simulink model "LDFIsys"  (R2023a)
settings: Solver=FixedStepDiscrete  StartTime=0.0  StopTime=cin.TimeInfo.End  RelTol=1e-3
values from neighbouring files (symbols this model uses):
  cmax = rows*cols    [LDFItest.m]    (also in LDXItest.m; LXFItest.m; LXFXtest.m; LXXItest.m)
  hmax = ceil((rows*cols/sqrt(12))/pow2(logDPS.stde,8-sbin))    [LDFItest.m]    (also in LDXItest.m; LXFItest.m; LXFXtest.m; LXXItest.m)
  sbin = 4    [LDFItest.m]    (also in LDXItest.m; LXFItest.m; LXFXtest.m; LXXItest.m)
  Ts = 1/(30*rows*cols)    [LDFItest.m]    (also in LDXItest.m; LXFItest.m; LXFXtest.m; LXXItest.m)
libraries: simulink x20, hdlsllib x5
settings Model: Creator=dileepan  LastModifiedBy=dileepan
settings DataIOCC: SaveOutput=off  SignalLogging=off  DSMLogging=off  SaveTime=off  ReturnWorkspaceOutputs=off

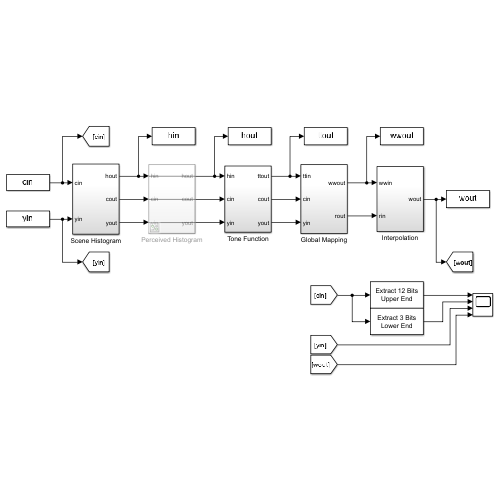
[thumbnail: Simulink's stored preview of the top-level diagram]
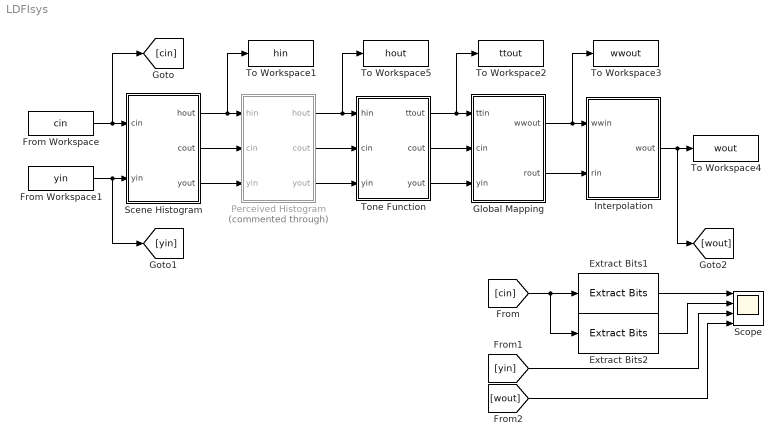
== system LDFIsys ==
  Extract Bits1 : simulink/Logic and Bit Operations/Extract Bits  bitsToExtract=Range starting with most significant bit  numBits=16-sbin  bitIdxRange=2+[0 15-sbin]  outScalingMode=Treat bit field as an integer
  Extract Bits2 : simulink/Logic and Bit Operations/Extract Bits  bitsToExtract=Range ending with least significant bit  numBits=3  bitIdxRange=[0 1]  outScalingMode=Treat bit field as an integer
  From Workspace : FromWorkspace  VariableName=cin  SampleTime=Ts  Interpolate=off  OutputAfterFinalValue=Setting to zero
  From Workspace1 : FromWorkspace  VariableName=yin  SampleTime=Ts  Interpolate=off  OutputAfterFinalValue=Setting to zero
  Global Mapping : Subsystem
  Interpolation : Subsystem
  Perceived Histogram : Subsystem  Commented=through
  Scene Histogram : Subsystem
  Scope : Scope  NumInputPorts=4
  To Workspace1 : ToWorkspace  VariableName=hin  SaveFormat=Timeseries  SampleTime=-1
      settings: Save2DSignal=2-D array (concatenate along first dimension)
  To Workspace2 : ToWorkspace  VariableName=ttout  SaveFormat=Timeseries  SampleTime=-1
      settings: Save2DSignal=2-D array (concatenate along first dimension)
  To Workspace3 : ToWorkspace  VariableName=wwout  SaveFormat=Timeseries  SampleTime=-1
      settings: Save2DSignal=2-D array (concatenate along first dimension)
  To Workspace4 : ToWorkspace  VariableName=wout  SaveFormat=Timeseries  SampleTime=-1
      settings: Save2DSignal=2-D array (concatenate along first dimension)
  To Workspace5 : ToWorkspace  VariableName=hout  SaveFormat=Timeseries  SampleTime=-1
      settings: Save2DSignal=2-D array (concatenate along first dimension)
  Tone Function : Subsystem
  wires:
  [cin] -> Extract Bits2/1, Extract Bits1/1
  Extract Bits1/1 -> Scope/1
  Extract Bits2/1 -> Scope/2
  [yin] -> Scope/3
  [wout] -> Scope/4
  Scene Histogram/3(yout) -> Perceived Histogram/3(yin)
  Scene Histogram/2(cout) -> Perceived Histogram/2(cin)
  Scene Histogram/1(hout) -> To Workspace1/1, Perceived Histogram/1(hin)
  Perceived Histogram/1(hout) -> To Workspace5/1, Tone Function/1(hin)
  Perceived Histogram/2(cout) -> Tone Function/2(cin)
  Perceived Histogram/3(yout) -> Tone Function/3(yin)
  Tone Function/1(ttout) -> To Workspace2/1, Global Mapping/1(ttin)
  Tone Function/2(cout) -> Global Mapping/2(cin)
  Tone Function/3(yout) -> Global Mapping/3(yin)
  Global Mapping/2(rout) -> Interpolation/2(rin)
  Global Mapping/1(wwout) -> To Workspace3/1, Interpolation/1(wwin)
  From Workspace/1 -> [cin], Scene Histogram/1(cin)
  Interpolation/1(wout) -> [wout], To Workspace4/1
  From Workspace1/1 -> [yin], Scene Histogram/2(yin)

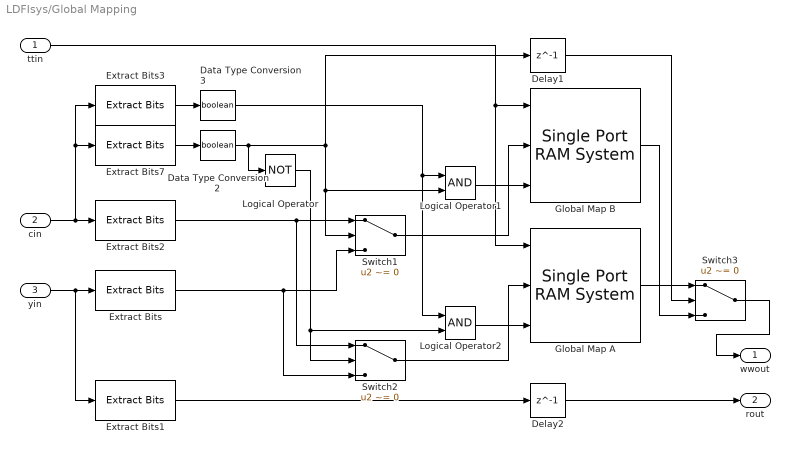
== system LDFIsys/Global Mapping ==
  ttin : Inport
  cin : Inport  Port=2
  yin : Inport  Port=3
  Data Type Conversion2 : DataTypeConversion  OutDataTypeStr=boolean  ConvertRealWorld=Stored Integer (SI)  SaturateOnIntegerOverflow=off  RndMeth=Floor
  Data Type Conversion3 : DataTypeConversion  OutDataTypeStr=boolean  ConvertRealWorld=Stored Integer (SI)  SaturateOnIntegerOverflow=off  RndMeth=Floor
  Delay1 : Delay  DelayLength=1
  Delay2 : Delay  DelayLength=1
  Extract Bits : simulink/Logic and Bit Operations/Extract Bits  bitsToExtract=Range starting with most significant bit  numBits=16-sbin  bitIdxRange=[0 7]  outScalingMode=Treat bit field as an integer
  Extract Bits1 : simulink/Logic and Bit Operations/Extract Bits  bitsToExtract=Range ending with least significant bit  numBits=sbin  bitIdxRange=0  outScalingMode=Treat bit field as an integer
  Extract Bits2 : simulink/Logic and Bit Operations/Extract Bits  bitsToExtract=Range starting with most significant bit  numBits=16-sbin  bitIdxRange=[2 17-sbin]  outScalingMode=Treat bit field as an integer
  Extract Bits3 : simulink/Logic and Bit Operations/Extract Bits  bitsToExtract=Range of bits  numBits=2  bitIdxRange=1  outScalingMode=Treat bit field as an integer
  Extract Bits7 : simulink/Logic and Bit Operations/Extract Bits  bitsToExtract=Range of bits  numBits=1  bitIdxRange=0  outScalingMode=Treat bit field as an integer
  Global Map A : hdlsllib/HDL RAMs/Single Port RAM System  RAMType=Single port  WriteOutputValue=New data  RAMInitialValue=0  SimulateUsing=Code generation
  Global Map B : hdlsllib/HDL RAMs/Single Port RAM System  RAMType=Single port  WriteOutputValue=New data  RAMInitialValue=0  SimulateUsing=Code generation
  Logical Operator : Logic  Operator=NOT  IconShape=distinctive  AllPortsSameDT=off  OutDataTypeStr=boolean
  Logical Operator1 : Logic  AllPortsSameDT=off  OutDataTypeStr=boolean
  Logical Operator2 : Logic  AllPortsSameDT=off  OutDataTypeStr=boolean
  Switch1 : Switch  Criteria=u2 ~= 0  SaturateOnIntegerOverflow=off  InputSameDT=off
  Switch2 : Switch  Criteria=u2 ~= 0  SaturateOnIntegerOverflow=off  InputSameDT=off
  Switch3 : Switch  Criteria=u2 ~= 0  SaturateOnIntegerOverflow=off  InputSameDT=off
  wwout : Outport
  rout : Outport  Port=2
  wires:
  yin/1 -> Extract Bits1/1, Extract Bits/1
  Extract Bits7/1 -> Data Type Conversion2/1
  Extract Bits/1 -> Switch2/3, Switch1/3
  Data Type Conversion3/1 -> Logical Operator1/1, Logical Operator2/1
  Switch1/1 -> Global Map B/2
  cin/1 -> Extract Bits2/1, Extract Bits3/1, Extract Bits7/1
  Extract Bits3/1 -> Data Type Conversion3/1
  Switch2/1 -> Global Map A/2
  Logical Operator/1 -> Logical Operator2/2, Switch2/2
  Extract Bits2/1 -> Switch2/1, Switch1/1
  Data Type Conversion2/1 -> Logical Operator/1, Delay1/1, Switch1/2, Logical Operator1/2
  Logical Operator1/1 -> Global Map B/3
  Logical Operator2/1 -> Global Map A/3
  Global Map A/1 -> Switch3/1
  Global Map B/1 -> Switch3/3
  ttin/1 -> Global Map B/1, Global Map A/1
  Extract Bits1/1 -> Delay2/1
  Delay2/1 -> rout/1
  Switch3/1 -> wwout/1
  Delay1/1 -> Switch3/2

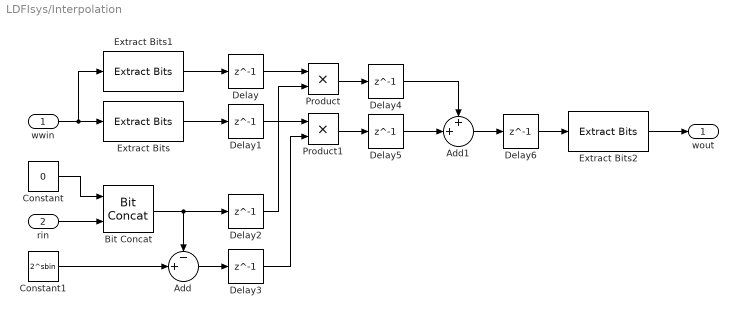
== system LDFIsys/Interpolation ==
  wwin : Inport
  rin : Inport  Port=2
  Add : Sum  Inputs=-+|  OutDataTypeStr=Inherit: Same as accumulator
  Add1 : Sum  Inputs=++|  OutDataTypeStr=Inherit: Same as accumulator
  Bit Concat : hdlsllib/Logic and Bit Operations/Bit Concat  numInputs=2
  Constant : Constant  Value=0  OutDataTypeStr=fixdt(0,1,0)  SampleTime=Ts
  Constant1 : Constant  Value=2^sbin  OutDataTypeStr=fixdt(0,sbin+1,0)  SampleTime=Ts
  Delay{,1..6} (7 alike) : Delay  DelayLength=1
  Extract Bits : simulink/Logic and Bit Operations/Extract Bits  bitsToExtract=Lower half  numBits=8  bitIdxRange=[0 7]  outScalingMode=Treat bit field as an integer
  Extract Bits1 : simulink/Logic and Bit Operations/Extract Bits  bitsToExtract=Upper half  numBits=8  bitIdxRange=[0 7]  outScalingMode=Treat bit field as an integer
  Extract Bits2 : simulink/Logic and Bit Operations/Extract Bits  bitsToExtract=Range of bits  numBits=8  bitIdxRange=[0 7]+sbin  outScalingMode=Treat bit field as an integer
  Product : Product  OutDataTypeStr=fixdt(0,8+sbin+1,0)
  Product1 : Product  OutDataTypeStr=fixdt(0,8+sbin+1,0)
  wout : Outport
  wires:
  wwin/1 -> Extract Bits1/1, Extract Bits/1
  rin/1 -> Bit Concat/2
  Constant/1 -> Bit Concat/1
  Extract Bits1/1 -> Delay/1
  Extract Bits/1 -> Delay1/1
  Bit Concat/1 -> Delay2/1, Add/1
  Delay2/1 -> Product/2
  Add/1 -> Delay3/1
  Delay3/1 -> Product1/2
  Delay/1 -> Product/1
  Delay1/1 -> Product1/1
  Product/1 -> Delay4/1
  Product1/1 -> Delay5/1
  Delay5/1 -> Add1/2
  Delay4/1 -> Add1/1
  Add1/1 -> Delay6/1
  Delay6/1 -> Extract Bits2/1
  Extract Bits2/1 -> wout/1
  Constant1/1 -> Add/2

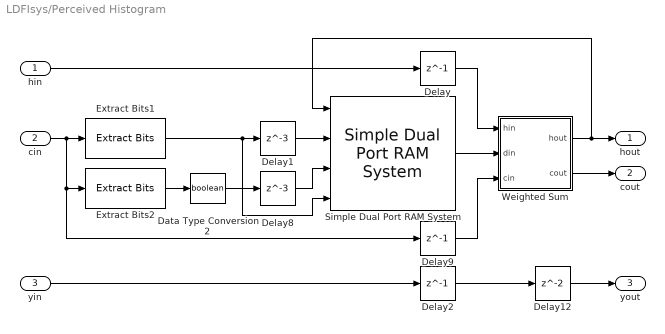
== system LDFIsys/Perceived Histogram ==
  hin : Inport
  cin : Inport  Port=2
  yin : Inport  Port=3
  Data Type Conversion2 : DataTypeConversion  OutDataTypeStr=boolean  ConvertRealWorld=Stored Integer (SI)  SaturateOnIntegerOverflow=off  RndMeth=Floor
  Delay : Delay  DelayLength=1
  Delay1 : Delay  DelayLength=3
  Delay12 : Delay
  Delay2 : Delay  DelayLength=1
  Delay8 : Delay  DelayLength=3
  Delay9 : Delay  DelayLength=1
  Extract Bits1 : simulink/Logic and Bit Operations/Extract Bits  bitsToExtract=Range starting with most significant bit  numBits=16-sbin  bitIdxRange=[3 18-sbin]  outScalingMode=Treat bit field as an integer
  Extract Bits2 : simulink/Logic and Bit Operations/Extract Bits  bitsToExtract=Range of bits  numBits=bitc  bitIdxRange=1  outScalingMode=Treat bit field as an integer
  Simple Dual Port RAM System : hdlsllib/HDL RAMs/Simple Dual Port RAM System  RAMType=Simple dual port  WriteOutputValue=New data  RAMInitialValue=0  SimulateUsing=Code generation
  Weighted Sum : Subsystem
  hout : Outport
  cout : Outport  Port=2
  yout : Outport  Port=3
  wires:
  hin/1 -> Delay/1
  Delay1/1 -> Simple Dual Port RAM System/2
  Extract Bits1/1 -> Simple Dual Port RAM System/4, Delay1/1
  cin/1 -> Delay9/1, Extract Bits2/1, Extract Bits1/1
  Delay8/1 -> Simple Dual Port RAM System/3
  yin/1 -> Delay2/1
  Delay12/1 -> yout/1
  Data Type Conversion2/1 -> Delay8/1
  Extract Bits2/1 -> Data Type Conversion2/1
  Simple Dual Port RAM System/1 -> Weighted Sum/2(din)
  Delay/1 -> Weighted Sum/1(hin)
  Delay9/1 -> Weighted Sum/3(cin)
  Delay2/1 -> Delay12/1
  Weighted Sum/1(hout) -> Simple Dual Port RAM System/1, hout/1
  Weighted Sum/2(cout) -> cout/1

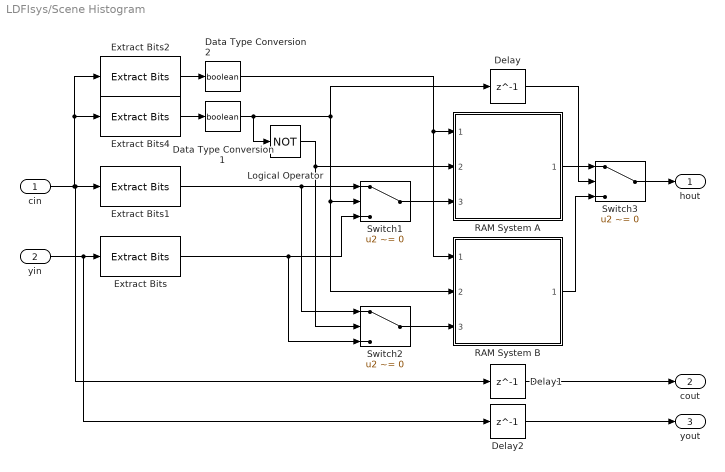
== system LDFIsys/Scene Histogram ==
  cin : Inport
  yin : Inport  Port=2
  Data Type Conversion1 : DataTypeConversion  OutDataTypeStr=boolean  ConvertRealWorld=Stored Integer (SI)  SaturateOnIntegerOverflow=off  RndMeth=Floor
  Data Type Conversion2 : DataTypeConversion  OutDataTypeStr=boolean  ConvertRealWorld=Stored Integer (SI)  SaturateOnIntegerOverflow=off  RndMeth=Floor
  Delay : Delay  DelayLength=1
  Delay1 : Delay  DelayLength=1
  Delay2 : Delay  DelayLength=1
  Extract Bits : simulink/Logic and Bit Operations/Extract Bits  bitsToExtract=Range starting with most significant bit  numBits=16-sbin  bitIdxRange=[0 7]  outScalingMode=Treat bit field as an integer
  Extract Bits1 : simulink/Logic and Bit Operations/Extract Bits  bitsToExtract=Range starting with most significant bit  numBits=16-sbin  bitIdxRange=[2 17-sbin]  outScalingMode=Treat bit field as an integer
  Extract Bits2 : simulink/Logic and Bit Operations/Extract Bits  bitsToExtract=Range of bits  numBits=2  bitIdxRange=1  outScalingMode=Treat bit field as an integer
  Extract Bits4 : simulink/Logic and Bit Operations/Extract Bits  bitsToExtract=Range of bits  numBits=1  bitIdxRange=0  outScalingMode=Treat bit field as an integer
  Logical Operator : Logic  Operator=NOT  IconShape=distinctive  AllPortsSameDT=off  OutDataTypeStr=boolean
  RAM System A : Subsystem  ReferencedSubsystem=RAMsys
  RAM System B : Subsystem  ReferencedSubsystem=RAMsys
  Switch1 : Switch  Criteria=u2 ~= 0  SaturateOnIntegerOverflow=off  InputSameDT=off
  Switch2 : Switch  Criteria=u2 ~= 0  SaturateOnIntegerOverflow=off  InputSameDT=off
  Switch3 : Switch  Criteria=u2 ~= 0  SaturateOnIntegerOverflow=off  InputSameDT=off
  hout : Outport
  cout : Outport  Port=2
  yout : Outport  Port=3
  wires:
  Extract Bits2/1 -> Data Type Conversion2/1
  Extract Bits/1 -> Switch2/3, Switch1/3
  yin/1 -> Delay2/1, Extract Bits/1
  Data Type Conversion1/1 -> Logical Operator/1, Delay/1, RAM System B/2, Switch1/2
  cin/1 -> Delay1/1, Extract Bits1/1, Extract Bits4/1, Extract Bits2/1
  Switch2/1 -> RAM System B/3
  Extract Bits1/1 -> Switch2/1, Switch1/1
  Logical Operator/1 -> Switch2/2, RAM System A/2
  Data Type Conversion2/1 -> RAM System B/1, RAM System A/1
  Extract Bits4/1 -> Data Type Conversion1/1
  Switch1/1 -> RAM System A/3
  Delay1/1 -> cout/1
  Delay2/1 -> yout/1
  Switch3/1 -> hout/1
  RAM System A/1 -> Switch3/1
  Delay/1 -> Switch3/2
  RAM System B/1 -> Switch3/3

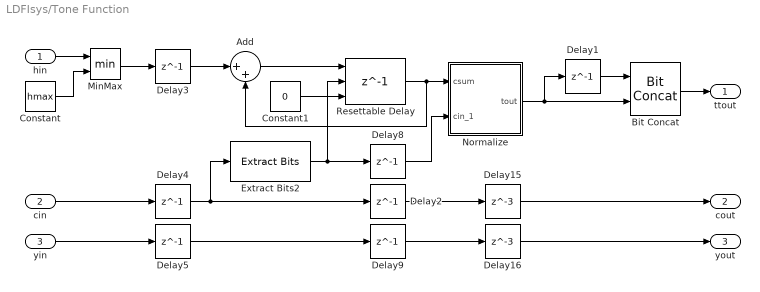
== system LDFIsys/Tone Function ==
  hin : Inport
  cin : Inport  Port=2
  yin : Inport  Port=3
  Add : Sum  Inputs=|++  OutDataTypeStr=Inherit: Same as accumulator
  Bit Concat : hdlsllib/Logic and Bit Operations/Bit Concat  numInputs=2
  Constant : Constant  Value=hmax  OutDataTypeStr=fixdt(0,ceil(log2(rows*cols)),0)  SampleTime=Ts
  Constant1 : Constant  Value=0  OutDataTypeStr=fixdt(0,bitc,0)  SampleTime=Ts
  Delay{1..5,8..9} (7 alike) : Delay  DelayLength=1
  Delay15 : Delay  DelayLength=3
  Delay16 : Delay  DelayLength=3
  Extract Bits2 : simulink/Logic and Bit Operations/Extract Bits  bitsToExtract=Range of bits  numBits=2  bitIdxRange=1  outScalingMode=Treat bit field as an integer
  MinMax : MinMax  Inputs=2
  Normalize : Subsystem
  Resettable Delay : Delay  DelayLength=1  InitialConditionSource=Input port  ExternalReset=Rising
      settings: InputPortMap=u0,r5,p4
  ttout : Outport
  cout : Outport  Port=2
  yout : Outport  Port=3
  wires:
  Extract Bits2/1 -> Resettable Delay/2, Delay8/1
  Delay15/1 -> cout/1
  Delay16/1 -> yout/1
  Bit Concat/1 -> ttout/1
  Delay1/1 -> Bit Concat/1
  Constant1/1 -> Resettable Delay/3
  Add/1 -> Resettable Delay/1
  hin/1 -> MinMax/1
  Constant/1 -> MinMax/2
  Resettable Delay/1 -> Normalize/1(csum), Add/2
  Delay9/1 -> Delay16/1
  Delay2/1 -> Delay15/1
  Delay8/1 -> Normalize/2(cin_1)
  Normalize/1(tout) -> Bit Concat/2, Delay1/1
  MinMax/1 -> Delay3/1
  Delay3/1 -> Add/1
  cin/1 -> Delay4/1
  Delay4/1 -> Delay2/1, Extract Bits2/1
  yin/1 -> Delay5/1
  Delay5/1 -> Delay9/1

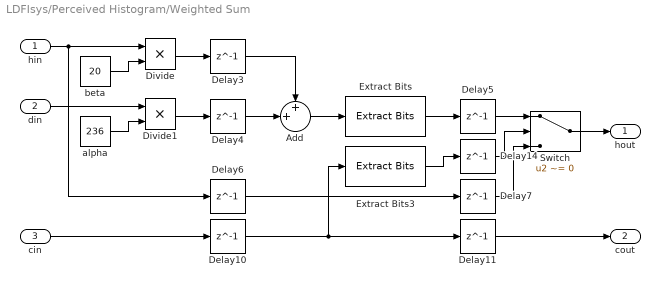
== system LDFIsys/Perceived Histogram/Weighted Sum ==
  hin : Inport
  din : Inport  Port=2
  cin : Inport  Port=3
  Add : Sum  Inputs=++|  OutDataTypeStr=Inherit: Same as accumulator
  Delay{3..7,10..11,14} (8 alike) : Delay  DelayLength=1
  Divide : Product  Inputs=**  OutDataTypeStr=fixdt(0,bitc+8,0)
  Divide1 : Product  Inputs=**  OutDataTypeStr=fixdt(0,bitc+8,0)
  Extract Bits : simulink/Logic and Bit Operations/Extract Bits  bitsToExtract=Range starting with most significant bit  numBits=bitc  bitIdxRange=[0 7]  outScalingMode=Treat bit field as an integer
  Extract Bits3 : simulink/Logic and Bit Operations/Extract Bits  bitsToExtract=Range of bits  numBits=bitc  bitIdxRange=2  outScalingMode=Treat bit field as an integer
  Switch : Switch  Criteria=u2 ~= 0  SaturateOnIntegerOverflow=off  InputSameDT=off
  alpha : Constant  Value=236  OutDataTypeStr=uint8  SampleTime=Ts
  beta : Constant  Value=20  OutDataTypeStr=uint8  SampleTime=Ts
  hout : Outport
  cout : Outport  Port=2
  wires:
  Delay5/1 -> Switch/1
  Divide/1 -> Delay3/1
  Delay4/1 -> Add/2
  Delay3/1 -> Add/1
  Divide1/1 -> Delay4/1
  cin/1 -> Delay10/1
  Delay6/1 -> Delay7/1
  Delay10/1 -> Extract Bits3/1, Delay11/1
  Extract Bits/1 -> Delay5/1
  Delay7/1 -> Switch/3
  Delay11/1 -> cout/1
  Extract Bits3/1 -> Delay14/1
  Delay14/1 -> Switch/2
  Add/1 -> Extract Bits/1
  Switch/1 -> hout/1
  hin/1 -> Delay6/1, Divide/1
  din/1 -> Divide1/1
  beta/1 -> Divide/2
  alpha/1 -> Divide1/2

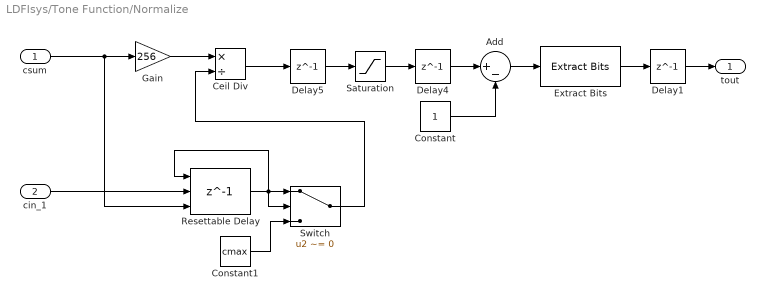
== system LDFIsys/Tone Function/Normalize ==
  csum : Inport
  cin_1 : Inport  Port=2
  Add : Sum  Inputs=|+-  OutDataTypeStr=Inherit: Same as accumulator
  Ceil Div : Product  Inputs=*/  OutDataTypeStr=fixdt(0,9,0)  RndMeth=Ceiling
  Constant : Constant  OutDataTypeStr=fixdt(0,1,0)  SampleTime=Ts
  Constant1 : Constant  Value=cmax  OutDataTypeStr=fixdt(0,bitc,0)  SampleTime=Ts
  Delay1 : Delay  DelayLength=1
  Delay4 : Delay  DelayLength=1
  Delay5 : Delay  DelayLength=1
  Extract Bits : simulink/Logic and Bit Operations/Extract Bits  bitsToExtract=Range ending with least significant bit  numBits=8  bitIdxRange=[0 7]  outScalingMode=Treat bit field as an integer
      settings: LibrarySourceBlock=|
      | hdlsllib/Logic and Bit
      | Operations/Extract Bits
  Gain : Gain  Gain=256  OutDataTypeStr=fixdt(0,bitc+8,0)
  Resettable Delay : Delay  DelayLength=1  InitialConditionSource=Input port  ExternalReset=Falling
      settings: InputPortMap=u0,r5,p4
  Saturation : Saturate  UpperLimit=256  LowerLimit=1
  Switch : Switch  Criteria=u2 ~= 0  SaturateOnIntegerOverflow=off  InputSameDT=off
  tout : Outport
  wires:
  Delay5/1 -> Saturation/1
  Ceil Div/1 -> Delay5/1
  Switch/1 -> Ceil Div/2
  Saturation/1 -> Delay4/1
  Resettable Delay/1 -> Switch/1, Switch/2, Resettable Delay/1
  Delay4/1 -> Add/1
  Extract Bits/1 -> Delay1/1
  Constant1/1 -> Switch/3
  Delay1/1 -> tout/1
  Gain/1 -> Ceil Div/1
  cin_1/1 -> Resettable Delay/2
  csum/1 -> Resettable Delay/3, Gain/1
  Constant/1 -> Add/2
  Add/1 -> Extract Bits/1
